simulink model "kurs_CE2018ok"  (R2019a)
settings: Solver=VariableStepAuto  StartTime=0.0  StopTime=0.1  RelTol=1e-3  EnableMultiTasking=on
libraries: powerlib x16, powerlib_extras x5
settings Model: Creator=MrCaoNhu  LastModifiedBy=ogure
settings DataIOCC: ReturnWorkspaceOutputs=off
settings OptimizationCC: LifeSpan=inf
settings DebuggingCC: SFUnexpectedBacktrackingDiag=warning  SFNoUnconditionalDefaultTransitionDiag=warning  ArithmeticOperatorsInVariantConditions=warning
settings SFSimCC: SimUseLocalCustomCode=off
settings RTWCC: RTWUseLocalCustomCode=off
settings CodeAppCC: StateflowObjectComments=on
settings GRTTargetCC: TargetLangStandard=C89/C90 (ANSI)  GeneratePreprocessorConditionals=Disable all
settings ConfigComp: CovMetricSettings=dw  CovHtmlReporting=on  CovSaveCumulativeToWorkspaceVar=on  CovSaveSingleToWorkspaceVar=on  CovExternalEMLEnable=off
settings SimscapeCC: SimscapeNormalizeSystem=off

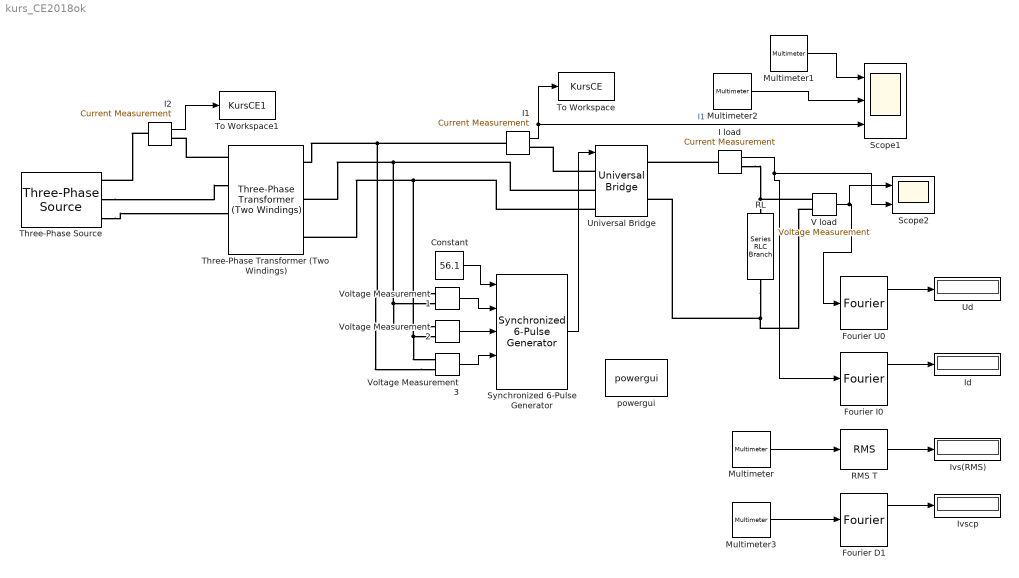
== system kurs_CE2018ok ==
  Constant : Constant  Value=56.1  VectorParams1D=off
  Fourier D1 : powerlib_extras/Measurements/Fourier  f1=50  n=0
      settings: SourceProductName=Simscape Electrical  SourceProductBaseCode=PS
  Fourier I0 : powerlib_extras/Measurements/Fourier  f1=300  n=0
      settings: SourceProductName=Simscape Electrical  SourceProductBaseCode=PS
  Fourier U0 : powerlib_extras/Measurements/Fourier  f1=300  n=0
      settings: SourceProductName=Simscape Electrical  SourceProductBaseCode=PS
  I load : powerlib/Measurements/Current Measurement  PhasorSimulation=off  OutputType=Complex  PSBequivalent=0
      settings: SourceProductName=Simscape Electrical
  I1 : powerlib/Measurements/Current Measurement  PhasorSimulation=off  OutputType=Complex  PSBequivalent=0
      settings: SourceProductName=Simscape Electrical
  I2 : powerlib/Measurements/Current Measurement  PhasorSimulation=off  OutputType=Complex  PSBequivalent=0
      settings: SourceProductName=Simscape Electrical
  Id : Display
      settings: Decimation=3
  Ivs(RMS) : Display
      settings: Decimation=3
  Ivsср : Display
      settings: Decimation=3
  Multimeter : powerlib/Measurements/Multimeter  PhasorSimulation=off  OutputType=Complex  sel=11  L=16  Gain=1  yselected={'Isw1: Universal Bridge'};  PSBOutputType=1  PSBequivalent=0  AxesSetting=[0,0.1,-100,100]  Display=0  SavedBlockNames=-11
      settings: SourceProductName=Simscape Electrical
  Multimeter1 : powerlib/Measurements/Multimeter  PhasorSimulation=off  OutputType=Complex  sel=[1 4]  L=16  Gain=[1 1]  yselected={'Usw1: Universal Bridge','Usw4: Universal Bridge'};  PSBOutputType=1  PSBequivalent=0  AxesSetting=[0,0.1,-100,100]  Display=0  SavedBlockNames=-11
      settings: SourceProductName=Simscape Electrical
  Multimeter2 : powerlib/Measurements/Multimeter  PhasorSimulation=off  OutputType=Complex  sel=[11 14]  L=16  Gain=[1 1]  yselected={'Isw1: Universal Bridge','Isw4: Universal Bridge'};  PSBOutputType=1  PSBequivalent=0  AxesSetting=[0,0.1,-100,100]  Display=0  SavedBlockNames=-11
      settings: SourceProductName=Simscape Electrical
  Multimeter3 : powerlib/Measurements/Multimeter  PhasorSimulation=off  OutputType=Complex  sel=11  L=16  Gain=1  yselected={'Isw1: Universal Bridge'};  PSBOutputType=1  PSBequivalent=0  AxesSetting=[0,0.1,-100,100]  Display=0  SavedBlockNames=-11
      settings: SourceProductName=Simscape Electrical
  RL : powerlib/Elements/Series RLC Branch  LConnTagsString=__new0  RConnTagsString=__new0  BranchType=RL  Resistance=0.04  Inductance=530.5e-6  SetiL0=off  InitialCurrent=0  Capacitance=inf  Setx0=off  InitialVoltage=0  Measurements=None
      settings: SourceProductName=Simscape Electrical
  RMS T : powerlib_extras/Measurements/RMS  f1=50
      settings: SourceProductName=Simscape Electrical  SourceProductBaseCode=PS
  Scope1 : Scope  NumInputPorts=3
  Scope2 : Scope  NumInputPorts=2
  Synchronized 6-Pulse Generator : powerlib_extras/Control  Blocks/Synchronized 6-Pulse Generator  freq=50  pwidth=10  Double_Pulse=off
      settings: SourceProductName=Simscape Electrical  SourceProductBaseCode=PS
  Three-Phase Transformer (Two Windings) : powerlib/Elements/Three-Phase Transformer (Two Windings)  Winding1Connection=Yn  Winding2Connection=Yg  CoreType=Three single-phase transformers  SetSaturation=off  Hysteresis=off  DataFile='hysteresis'  SetInitialFlux=off  Measurements=None  UNITS=pu  NominalPower=[ 20e3 , 50 ]  Winding1=[ 230*sqrt(3) , 0.0 , 0.00 ]  Winding2=[ 8.2*sqrt(3) , 00 , 0 ]  Rm=500  Lm=500  L0=0.5  Saturation=[ 0,0 ; 0.0024,1.2 ; 1.0,1.52 ]  InitialFluxes=[ 0.8 , -0.8 , 0.7 ]  BreakLoop=off  DiscreteSolver=Trapezoidal iterative  DataType=off  TransfoNumber=1
      settings: SourceProductName=Simscape Electrical
  Three-Phase Source : powerlib/Electrical Sources/Three-Phase Source  InternalConnection=Yn  VoltagePhases=off  Voltage=320*sqrt(3)  PhaseAngle=0  Voltage_phases=[25e3 25e3 25e3]/sqrt(3)  PhaseAngles_phases=[0 -120 +120]  Frequency=50  NonIdealSource=off  SpecifyImpedance=off  Resistance=0.0156  Inductance=5.205*10^-5  ShortCircuitLevel=100e6  BaseVoltage=25e3  XRratio=7  BusType=swing  Pref=0  Qref=0  Prefabc=[10e3, 10e3, 10e3]  Qrefabc=[0, 0, 0]  Qmin=-inf  Qmax=inf
      settings: SourceProductName=Simscape Electrical
  To Workspace : ToWorkspace  VariableName=KursCE  SampleTime=2e-4
      settings: MaxDataPoints=200
  To Workspace1 : ToWorkspace  VariableName=KursCE1  SampleTime=2e-4
      settings: MaxDataPoints=200
  Ud : Display
      settings: Decimation=3
  Universal Bridge : powerlib/Power Electronics/Universal Bridge  Arms=3  SnubberResistance=1e6  SnubberCapacitance=1e-9  Device=Thyristors  Ron=1.05e-3  Lon=0  ForwardVoltages="[  0  0  ]"  ForwardVoltage=1.05  GTOparameters=[ 10e-6 , 20e-6 ]  IGBTparameters=[ 1e-6 , 2e-6 ]  Measurements=All voltages and currents  Measurements_2=None  converterType=Rectifier
      settings: SourceProductName=Simscape Electrical
  V load : powerlib/Measurements/Voltage Measurement  PhasorSimulation=off  OutputType=Complex  PSBequivalent=0
      settings: SourceProductName=Simscape Electrical
  Voltage Measurement1 : powerlib/Measurements/Voltage Measurement  PhasorSimulation=off  OutputType=Complex  PSBequivalent=0
      settings: SourceProductName=Simscape Electrical
  Voltage Measurement2 : powerlib/Measurements/Voltage Measurement  PhasorSimulation=off  OutputType=Complex  PSBequivalent=0
      settings: SourceProductName=Simscape Electrical
  Voltage Measurement3 : powerlib/Measurements/Voltage Measurement  PhasorSimulation=off  OutputType=Complex  PSBequivalent=0
      settings: SourceProductName=Simscape Electrical
  powergui : powerlib/powergui  Priority=1  SimulationMode=Discrete  SampleTime=1e-5  frequency=60  Iterations=50  frequencyindice=50  Pbase=100e6  ErrMax=1e-4  UnitsV=kV  UnitsW=MW  buscounter=0  FunctionMessages=off  echomessages=off  EnableUseOfTLC=off  CurrentSourceSwitches=on  DisableSnubberDevices=off  DisableRonSwitches=off  DisableVfSwitches=off  DisplayEquations=off  AutomaticDiscreteSolvers=off  SolverType=Tustin/Backward Euler (TBE)  Interpol=off  ExternalGateDelay=off  methode=off  Ts=100  x0status=blocks  SPID=off  SwTol=0  HookPort=off  NonlinearTolerance=0  nMaxIteration=15  ContinueOnMaxIteration=off  RestoreLinks=warning  ResistiveCurrentMeasurement=off  Frange=[0:2:500]  Ylog=off  Xlog=on  ShowGrid=off  save=off  variable=ZData  structure=0  ZoomFFT=off  StartTime=0.0  cycles=1  DisplayStyle=1  fundamental=60  FreqAxis=off  MaxFrequency=1000  frequencyindicesteady=1  RmsSteady=1  display=off
      settings: SourceProductName=Simscape Electrical
  wires:
  Voltage Measurement1/1 -> Synchronized 6-Pulse Generator/2
  Voltage Measurement2/1 -> Synchronized 6-Pulse Generator/3
  Voltage Measurement3/1 -> Synchronized 6-Pulse Generator/4
  Constant/1 -> Synchronized 6-Pulse Generator/1
  Synchronized 6-Pulse Generator/1 -> Universal Bridge/1
  I1/1 -> To Workspace/1, Scope1/3  "I1"
  I2/1 -> To Workspace1/1
  RMS T/1 -> Ivs(RMS)/1
  Multimeter/1 -> RMS T/1
  Fourier U0/1 -> Ud/1
  V load/1 -> Scope2/1, Fourier U0/1
  Fourier D1/1 -> Ivsср/1
  Multimeter3/1 -> Fourier D1/1
  Fourier I0/1 -> Id/1
  I load/1 -> Scope2/2, Fourier I0/1
  Multimeter1/1 -> Scope1/1
  Multimeter2/1 -> Scope1/2
  connections:
  I2/LConn1 -- Three-Phase Source/RConn1
  Three-Phase Source/RConn2 -- Three-Phase Transformer (Two Windings)/LConn2
  Three-Phase Source/RConn3 -- Three-Phase Transformer (Two Windings)/LConn3
  Voltage Measurement2/LConn1 -- Voltage Measurement1/LConn2 -- Three-Phase Transformer (Two Windings)/RConn2 -- Universal Bridge/LConn2
  Universal Bridge/LConn3 -- Three-Phase Transformer (Two Windings)/RConn3 -- Voltage Measurement2/LConn2 -- Voltage Measurement3/LConn1
  RL/LConn1 -- I load/RConn1 -- V load/LConn1
  Universal Bridge/RConn2 -- RL/RConn1 -- V load/LConn2
  Universal Bridge/LConn1 -- I1/RConn1
  I load/LConn1 -- Universal Bridge/RConn1
  Voltage Measurement3/LConn2 -- Three-Phase Transformer (Two Windings)/RConn1 -- I1/LConn1 -- Voltage Measurement1/LConn1
  Three-Phase Transformer (Two Windings)/LConn1 -- I2/RConn1
